simulink model "FixedWing_Linear_Sim"  (R2019b)
settings: Solver=ode5  StartTime=0.0  StopTime=10.0  FixedStep=0.01  RelTol=1e-3
values from neighbouring files (symbols this model uses):
  A_Lat = A(5:8, 5:8)    [FixedWing_Linear_Audit.m]
  a_lin = 0    [FixedWing_Linear_Audit.m]
  A_Long = A(1:4, 1:4)    [FixedWing_Linear_Audit.m]
  B_Lat = B(5:8, 2:3)    [FixedWing_Linear_Audit.m]
  B_Long = B(1:4, 1)    [FixedWing_Linear_Audit.m]
  C_Lat = C(5:8, 5:8)    [FixedWing_Linear_Audit.m]
  C_Long = C(1:4, 1:4)    [FixedWing_Linear_Audit.m]
  D_Lat = D(5:8, 2:3)    [FixedWing_Linear_Audit.m]
  D_Long = D(1:4, 1)    [FixedWing_Linear_Audit.m]
  e_lin = 0    [FixedWing_Linear_Audit.m]
  r_lin = -2.0 * d2r    [FixedWing_Linear_Audit.m]
undefined symbols (not defined in the file or in its folder): r2d
settings Model: Creator=peter  LastModifiedBy=peter

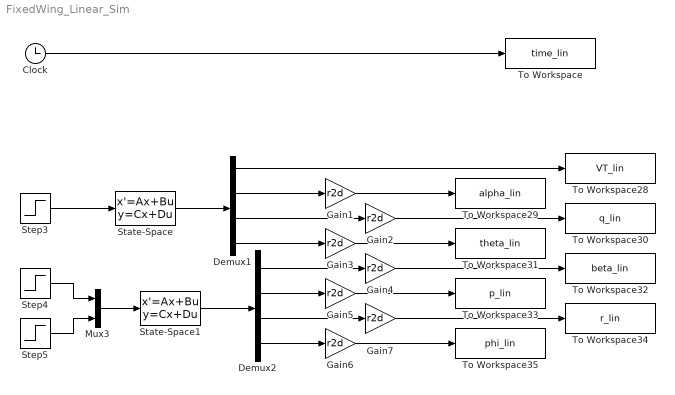
== system FixedWing_Linear_Sim ==
  Clock : Clock
  Demux1 : Demux
  Demux2 : Demux
  Gain{1..7} (7 alike) : Gain  Gain=r2d
  Mux3 : Mux  Inputs=2
  State-Space : StateSpace  A=A_Long  B=B_Long  C=C_Long  D=D_Long  InitialCondition=0
  State-Space1 : StateSpace  A=A_Lat  B=B_Lat  C=C_Lat  D=D_Lat  InitialCondition=0
  Step3 : Step  After=e_lin  SampleTime=0
  Step4 : Step  After=a_lin  SampleTime=0
  Step5 : Step  After=r_lin  SampleTime=0
  To Workspace : ToWorkspace  VariableName=time_lin  SampleTime=-1
  To Workspace28 : ToWorkspace  VariableName=VT_lin  SampleTime=-1
  To Workspace29 : ToWorkspace  VariableName=alpha_lin  SampleTime=-1
  To Workspace30 : ToWorkspace  VariableName=q_lin  SampleTime=-1
  To Workspace31 : ToWorkspace  VariableName=theta_lin  SampleTime=-1
  To Workspace32 : ToWorkspace  VariableName=beta_lin  SampleTime=-1
  To Workspace33 : ToWorkspace  VariableName=p_lin  SampleTime=-1
  To Workspace34 : ToWorkspace  VariableName=r_lin  SampleTime=-1
  To Workspace35 : ToWorkspace  VariableName=phi_lin  SampleTime=-1
  wires:
  Demux1/3 -> Gain2/1
  Demux2/1 -> Gain4/1
  Demux2/3 -> Gain7/1
  Step3/1 -> State-Space/1
  State-Space1/1 -> Demux2/1
  State-Space/1 -> Demux1/1
  Demux2/4 -> Gain6/1
  Step5/1 -> Mux3/2
  Demux2/2 -> Gain5/1
  Demux1/4 -> Gain3/1
  Mux3/1 -> State-Space1/1
  Demux1/2 -> Gain1/1
  Step4/1 -> Mux3/1
  Clock/1 -> To Workspace/1
  Demux1/1 -> To Workspace28/1
  Gain1/1 -> To Workspace29/1
  Gain2/1 -> To Workspace30/1
  Gain3/1 -> To Workspace31/1
  Gain4/1 -> To Workspace32/1
  Gain5/1 -> To Workspace33/1
  Gain7/1 -> To Workspace34/1
  Gain6/1 -> To Workspace35/1
